simulink model "esercitazione2"  (R2023b)
settings: Solver=VariableStepAuto  StartTime=0.0  StopTime=1200  MaxStep=0.01  RelTol=1e-3
InitFcn:
  | init2
values from neighbouring files (symbols this model uses):
  I = [I_x; I_y; I_z]    [init2.m]
  qi = [1; 0; 0; 0]    [init2.m]
  w_ic = [0; -w_o; 0]    [init2.m]
settings Model: Creator=dario  LastModifiedBy=dario

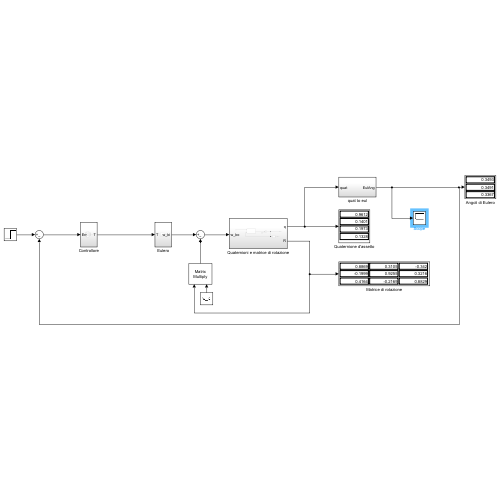
[thumbnail: Simulink's stored preview of the top-level diagram]
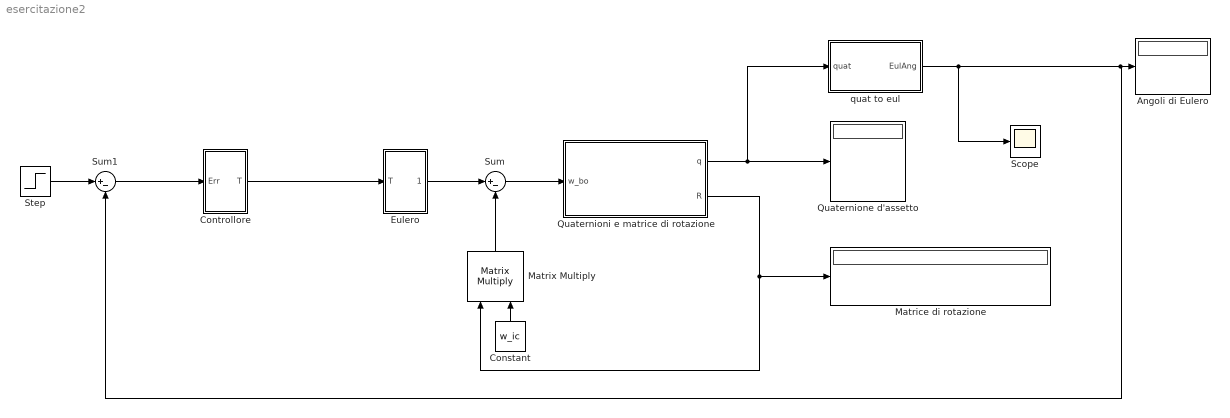
== system esercitazione2 ==
  Angoli di Eulero : Display
  Constant : Constant  Value=w_ic  VectorParams1D=off
  Controllore : Subsystem
  Eulero : Subsystem
  Matrice di rotazione : Display
  Matrix Multiply : Product  Inputs=**  Multiplication=Matrix(*)
  Quaternione d'assetto : Display
  Quaternioni e matrice di rotazione : Subsystem
  Scope : Scope
  Step : Step  After=20*pi/180  SampleTime=0  VectorParams1D=off
  Sum : Sum  Inputs=|+-
  Sum1 : Sum  Inputs=|+-
  quat to eul : Subsystem
  wires:
  Constant/1 -> Matrix Multiply/2
  Matrix Multiply/1 -> Sum/2
  Eulero/1(w_bi) -> Sum/1
  Quaternioni e matrice di rotazione/2(R) -> Matrix Multiply/1, Matrice di rotazione/1
  Sum/1 -> Quaternioni e matrice di rotazione/1(w_bo)
  Quaternioni e matrice di rotazione/1(q) -> quat to eul/1(quat), Quaternione d'assetto/1
  quat to eul/1(EulAng) -> Sum1/2, Angoli di Eulero/1, Scope/1
  Step/1 -> Sum1/1
  Sum1/1 -> Controllore/1(Err)
  Controllore/1(T) -> Eulero/1(T)

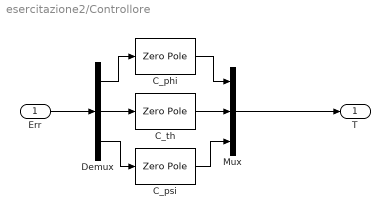
== system esercitazione2/Controllore ==
  Err : Inport
  C_phi : ZeroPole  Zeros=[-0.00275570824833914]  Poles=[-18.7954391846556]  Gain=0.3003
  C_psi : ZeroPole  Zeros=[-0.000562922792010666]  Poles=[-0.542363985961437]  Gain=5.615452434806354e-04
  C_th : ZeroPole  Zeros=[-0.0506603134003083]  Poles=[-4.40176222937419]  Gain=0.115928251260689
  Demux : Demux  Outputs=3
  Mux : Mux  Inputs=3
  T : Outport
  wires:
  Demux/1 -> C_phi/1
  C_th/1 -> Mux/2
  C_psi/1 -> Mux/3
  Demux/3 -> C_psi/1
  Err/1 -> Demux/1
  Demux/2 -> C_th/1
  C_phi/1 -> Mux/1
  Mux/1 -> T/1

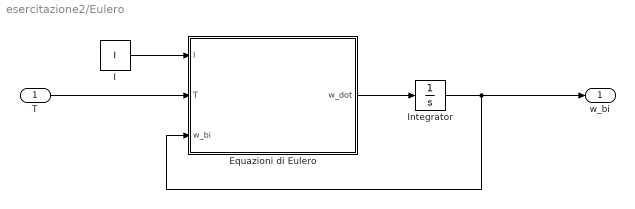
== system esercitazione2/Eulero ==
  T : Inport
  Equazioni di Eulero : MATLAB Function  TreatAsAtomicUnit=on
  I : Constant  Value=I  VectorParams1D=off
  Integrator : Integrator  InitialCondition=w_ic
  w_bi : Outport
  wires:
  I/1 -> Equazioni di Eulero/1(I)
  Equazioni di Eulero/1(w_dot) -> Integrator/1
  Integrator/1 -> w_bi/1, Equazioni di Eulero/3(w_bi)
  T/1 -> Equazioni di Eulero/2(T)

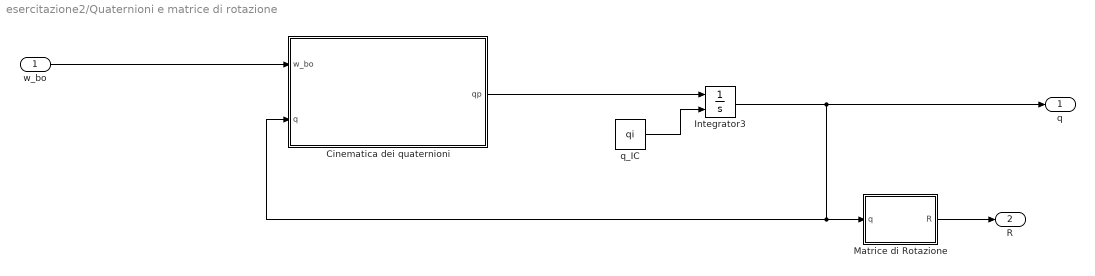
== system esercitazione2/Quaternioni e matrice di rotazione ==
  w_bo : Inport
  Cinematica dei quaternioni : MATLAB Function  TreatAsAtomicUnit=on
  Integrator3 : Integrator  InitialConditionSource=external
  Matrice di Rotazione : MATLAB Function  TreatAsAtomicUnit=on
  q_IC : Constant  Value=qi  VectorParams1D=off
  q : Outport
  R : Outport  Port=2
  wires:
  Integrator3/1 -> q/1, Cinematica dei quaternioni/2(q), Matrice di Rotazione/1(q)
  q_IC/1 -> Integrator3/2
  Matrice di Rotazione/1(R) -> R/1
  Cinematica dei quaternioni/1(qp) -> Integrator3/1
  w_bo/1 -> Cinematica dei quaternioni/1(w_bo)

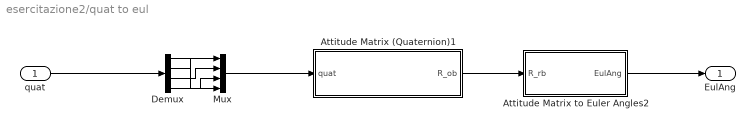
== system esercitazione2/quat to eul ==
  quat : Inport
  Attitude Matrix (Quaternion)1 : Subsystem
  Attitude Matrix to Euler Angles2 : Subsystem
  Demux : Demux
  Mux : Mux
  EulAng : Outport  VectorParamsAs1DForOutWhenUnconnected=off
  wires:
  Attitude Matrix to Euler Angles2/1(EulAng) -> EulAng/1
  Attitude Matrix (Quaternion)1/1(R_ob) -> Attitude Matrix to Euler Angles2/1(R_rb)
  quat/1 -> Demux/1
  Mux/1 -> Attitude Matrix (Quaternion)1/1(quat)
  Demux/1 -> Mux/4
  Demux/2 -> Mux/1
  Demux/3 -> Mux/2
  Demux/4 -> Mux/3

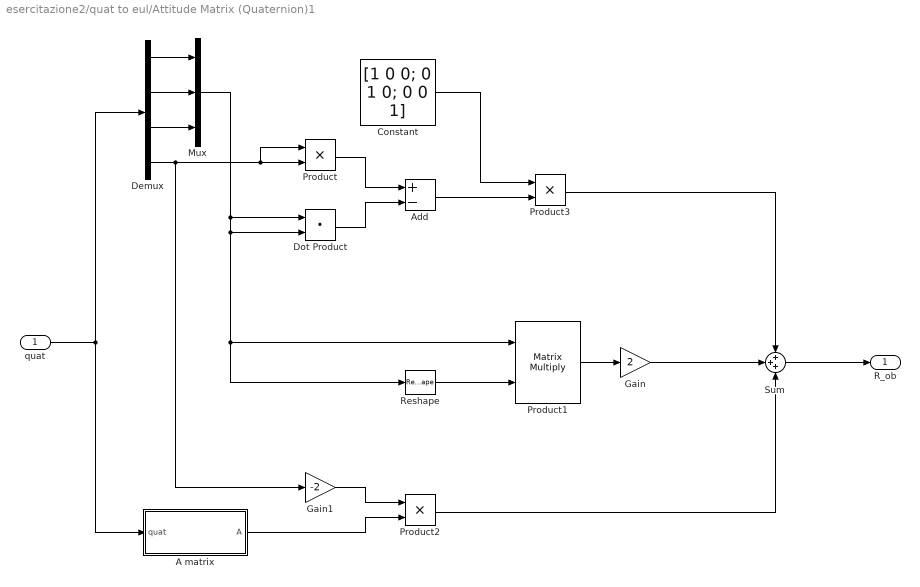
== system esercitazione2/quat to eul/Attitude Matrix (Quaternion)1 ==
  quat : Inport
  A matrix : Subsystem
  Add : Sum  Inputs=+-
  Constant : Constant  Value=[1 0 0; 0 1 0; 0 0 1]
  Demux : Demux
  Dot Product : DotProduct  OutDataTypeStr=Inherit: Inherit via internal rule
  Gain : Gain  Gain=2
  Gain1 : Gain  Gain=-2
  Mux : Mux  Inputs=3
  Product : Product  RndMeth=Zero
  Product1 : Product  Multiplication=Matrix(*)  RndMeth=Zero
  Product2 : Product  RndMeth=Zero
  Product3 : Product  RndMeth=Zero
  Reshape : Reshape  OutputDimensionality=Row vector (2-D)
  Sum : Sum  Inputs=+++
  R_ob : Outport  VectorParamsAs1DForOutWhenUnconnected=off
  wires:
  quat/1 -> Demux/1, A matrix/1(quat)
  Demux/4 -> Product/2, Product/1, Gain1/1
  Reshape/1 -> Product1/2
  Product1/1 -> Gain/1
  Gain/1 -> Sum/2
  Product/1 -> Add/1
  Dot Product/1 -> Add/2
  Product2/1 -> Sum/3
  Add/1 -> Product3/2
  Sum/1 -> R_ob/1
  Constant/1 -> Product3/1
  Product3/1 -> Sum/1
  Demux/1 -> Mux/1
  Demux/2 -> Mux/2
  Demux/3 -> Mux/3
  Mux/1 -> Dot Product/1, Reshape/1, Product1/1, Dot Product/2
  Gain1/1 -> Product2/1
  A matrix/1(A) -> Product2/2

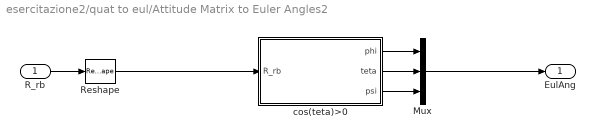
== system esercitazione2/quat to eul/Attitude Matrix to Euler Angles2 ==
  R_rb : Inport
  Mux : Mux  Inputs=3
  Reshape : Reshape  OutputDimensionality=Column vector (2-D)
  cos(teta)>0 : Subsystem
  EulAng : Outport  VectorParamsAs1DForOutWhenUnconnected=off
  wires:
  cos(teta)>0/2(teta) -> Mux/2
  cos(teta)>0/1(phi) -> Mux/1
  cos(teta)>0/3(psi) -> Mux/3
  Mux/1 -> EulAng/1
  Reshape/1 -> cos(teta)>0/1(R_rb)
  R_rb/1 -> Reshape/1

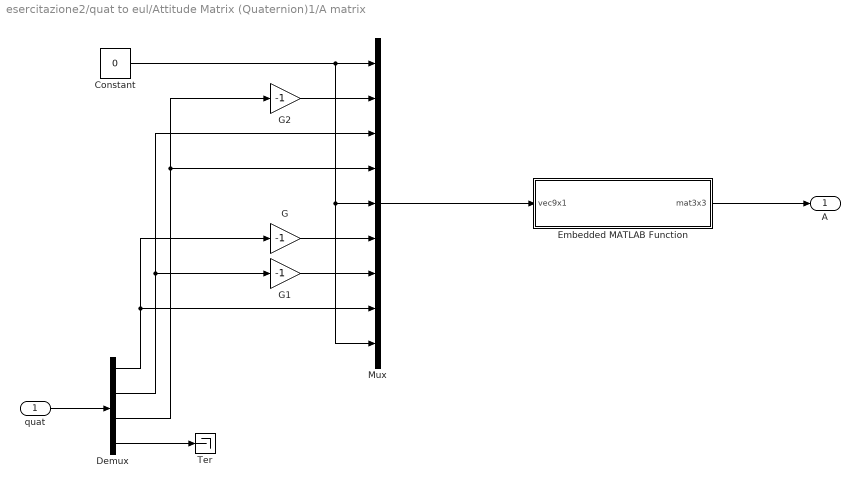
== system esercitazione2/quat to eul/Attitude Matrix (Quaternion)1/A matrix ==
  quat : Inport
  Constant : Constant  Value=0
  Demux : Demux
  Embedded MATLAB Function : MATLAB Function  TreatAsAtomicUnit=on
  G : Gain  Gain=-1
  G1 : Gain  Gain=-1
  G2 : Gain  Gain=-1
  Mux : Mux  Inputs=9
  Ter : Terminator
  A : Outport  VectorParamsAs1DForOutWhenUnconnected=off
  wires:
  Demux/4 -> Ter/1
  quat/1 -> Demux/1
  Constant/1 -> Mux/9, Mux/5, Mux/1
  Demux/1 -> G/1, Mux/8
  G1/1 -> Mux/7
  Demux/2 -> G1/1, Mux/3
  G/1 -> Mux/6
  G2/1 -> Mux/2
  Demux/3 -> G2/1, Mux/4
  Embedded MATLAB Function/1(mat3x3) -> A/1
  Mux/1 -> Embedded MATLAB Function/1(vec9x1)

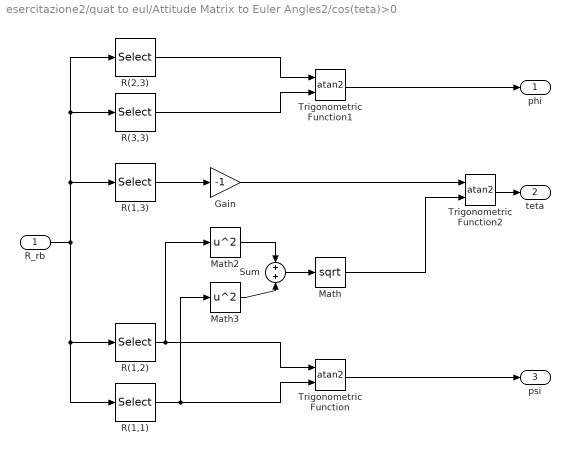
== system esercitazione2/quat to eul/Attitude Matrix to Euler Angles2/cos(teta)>0 ==
  R_rb : Inport
  Gain : Gain  Gain=-1
  Math : Math  Operator=sqrt  SignedPower=on
  Math2 : Math  Operator=square  SignedPower=on
  Math3 : Math  Operator=square  SignedPower=on
  R(1,1) : Selector  InputPortWidth=9  IndexOptions=Index vector (dialog)  Indices=[1]  OutputSizes=1
  R(1,2) : Selector  InputPortWidth=9  IndexOptions=Index vector (dialog)  Indices=[4]  OutputSizes=1
  R(1,3) : Selector  InputPortWidth=9  IndexOptions=Index vector (dialog)  Indices=[7]  OutputSizes=1
  R(2,3) : Selector  InputPortWidth=9  IndexOptions=Index vector (dialog)  Indices=[8]  OutputSizes=1
  R(3,3) : Selector  InputPortWidth=9  IndexOptions=Index vector (dialog)  Indices=[9]  OutputSizes=1
  Sum : Sum
  Trigonometric Function : Trigonometry  Operator=atan2
  Trigonometric Function1 : Trigonometry  Operator=atan2
  Trigonometric Function2 : Trigonometry  Operator=atan2
  phi : Outport  VectorParamsAs1DForOutWhenUnconnected=off
  teta : Outport  Port=2  VectorParamsAs1DForOutWhenUnconnected=off
  psi : Outport  Port=3  VectorParamsAs1DForOutWhenUnconnected=off
  wires:
  R_rb/1 -> R(1,1)/1, R(1,2)/1, R(1,3)/1, R(3,3)/1, R(2,3)/1
  R(1,2)/1 -> Trigonometric Function/1, Math2/1
  R(1,1)/1 -> Trigonometric Function/2, Math3/1
  R(2,3)/1 -> Trigonometric Function1/1
  R(3,3)/1 -> Trigonometric Function1/2
  R(1,3)/1 -> Gain/1
  Gain/1 -> Trigonometric Function2/1
  Math2/1 -> Sum/1
  Math3/1 -> Sum/2
  Sum/1 -> Math/1
  Math/1 -> Trigonometric Function2/2
  Trigonometric Function1/1 -> phi/1
  Trigonometric Function2/1 -> teta/1
  Trigonometric Function/1 -> psi/1

== matlab function esercitazione2/Quaternioni e matrice di rotazione/Cinematica dei quaternioni ==
  data: w_bo input; qp output; q input
function qp = Quaternioni(w_bo,q)
w_box=w_bo(1);
w_boy=w_bo(2);
w_boz=w_bo(3);

Q=[0 -w_box -w_boy -w_boz;
    w_box 0 w_boz -w_boy; 
    w_boy -w_boz 0 w_box; 
    w_boz w_boy -w_box 0];

qp=0.5*Q*q;

== matlab function esercitazione2/Eulero/Equazioni di Eulero ==
  data: I input; w_dot output; T input; w_bi input
function w_dot = Eulero(I,T,w_bi)
I_x=I(1);
I_y=I(2);
I_z=I(3);
T_x=T(1);
T_y=T(2);
T_z=T(3);
w_bix=w_bi(1);
w_biy=w_bi(2);
w_biz=w_bi(3);
a_x=-w_biy*w_biz*((I_z-I_y)/(I_x))+T_x/I_x;
a_y=-w_bix*w_biz*((I_x-I_z)/(I_y))+T_y/I_y;
a_z=-w_bix*w_biy*((I_y-I_x)/(I_z))+T_z/I_z;

w_dot=[a_x;a_y;a_z];

== matlab function esercitazione2/Quaternioni e matrice di rotazione/Matrice di Rotazione ==
  data: q input; R output
function R = rotmat(q)
i=eye(3);
qdir=[q(2); q(3); q(4)];
A=[0 -q(4) q(3); q(4) 0 -q(2); -q(3) q(2) 0];
R=(q(1)^2-dot(qdir,qdir))*i+2*(qdir*qdir')-2*q(1)*A;

== matlab function esercitazione2/quat to eul/Attitude Matrix (Quaternion)1/A matrix/Embedded MATLAB Function ==
  data: vec9x1 input; mat3x3 output
function mat3x3 = vec2mat(vec9x1)
%#eml

s = size(vec9x1);

if s(1)>s(2)
    vec = vec9x1';
else
    vec = vec9x1;
end

mat3x3 = [vec(1:3); vec(4:6); vec(7:9)];
